simulink model "ModeAdjust"  (R2018b)
settings: Solver=FixedStepDiscrete  StartTime=0.0  StopTime=inf  FixedStep=0.01  RelTol=1e-3
undefined symbols (not defined in the file or in its folder): IfKeSMSbSeatMovBkRclnEnable_Val, IfKeSMSbSeatMovFrwdBkwdEnable_Val, IfKeSMSbSeatMovFtrstEnable_Val, IfKeSMSbSeatMovHdrstFrwdBkwdEnable_Val, IfKeSMSbSeatMovHdUpwdDnwdEnable_Val, IfKeSMSbSeatMovLgrstEnable_Val, IfKeSMSbSeatMovLtwdRtwdEnable_Val, IfVeSMSeStNumConfig, KeSMSbArmscreenMovEnable_Val, KeSMSbSeatMovLgrstExpdEnable_Val, KeSMSuFirstRwStBackPosDelta_Val, KeSMSuFirstRwStBackPosTolr_Val, KeSMSuFirstRwStCushFrntPosDelta_Val, KeSMSuFirstRwStCushFrntPosTolr_Val, KeSMSuFirstRwStCushRePosDelta_Val, KeSMSuFirstRwStCushRePosTolr_Val, KeSMSuFirstRwStFootrestPosDelta_Val, KeSMSuFirstRwStFootrestPosTolr_Val, KeSMSuFirstRwStFwdBkwdPosDelta_Val, KeSMSuFirstRwStFwdBkwdPosTolr_Val, KeSMSuMdMotFinshdTm_Val, KeSMSuMdRetryTm1_Val, KeSMSuModeReqDurgTm_Val, KeSMSuSecRwStArmTochPosDelta_Val, KeSMSuSecRwStArmTochPosTolr_Val, KeSMSuSecRwStBackPosDelta_Val, KeSMSuSecRwStBackPosTolr_Val, KeSMSuSecRwStFtrstUpwdDnwdPosDelta_Val, KeSMSuSecRwStFtrstUpwdDnwdPosTolr_Val, KeSMSuSecRwStFwdBkwdPosDelta_Val, KeSMSuSecRwStFwdBkwdPosTolr_Val, KeSMSuSecRwStHeadrestFwdBkwdPosDelta_Val, KeSMSuSecRwStHeadrestFwdBkwdPosTolr_Val, KeSMSuSecRwStHeadrestUpwdDwnwdPosDelta_Val, KeSMSuSecRwStHeadrestUpwdDwnwdPosTolr_Val, KeSMSuSecRwStLegrestInOutPosDelta_Val, KeSMSuSecRwStLegrestInOutPosTolr_Val, KeSMSuSecRwStLegrestUpwdDwnwdPosDelta_Val, KeSMSuSecRwStLegrestUpwdDwnwdPosTolr_Val, KeSMSuSecRwStLwdRwdPosDelta_Val, KeSMSuSecRwStLwdRwdPosTolr_Val, KeSMSuSecRwStVIPFtrstRefAngle_Val, KeSMSuThirdRwStFwdBkwdPosDelta_Val, KeSMSuThirdRwStFwdBkwdPosTolr_Val, KeSMSuThrdRwCushFoldPosDelta_Val, KeSMSuThrdRwCushFoldPosTolr_Val, KeSMSuThrdRwStBackPosDelta_Val, KeSMSuThrdRwStBackPosTolr_Val, KeSMSw4SLegrstCloseMdSecRwLtStFtrstUpwdDnwdPos_Val, KeSMSw4SLegrstCloseMdSecRwLtStFtrstUpwdDnwdPosMax_Val, KeSMSw4SLegrstCloseMdSecRwLtStFtrstUpwdDnwdPosMin_Val, KeSMSw4SLegrstCloseMdSecRwLtStLgrstOtwdInwdPos_Val, KeSMSw4SLegrstCloseMdSecRwLtStLgrstOtwdInwdPosMax_Val, KeSMSw4SLegrstCloseMdSecRwLtStLgrstOtwdInwdPosMin_Val, KeSMSw4SLegrstCloseMdSecRwLtStLgrstUpwdDnwdPos_Val, KeSMSw4SLegrstCloseMdSecRwLtStLgrstUpwdDnwdPosMax_Val, KeSMSw4SLegrstCloseMdSecRwLtStLgrstUpwdDnwdPosMin_Val, KeSMSw4SLegrstCloseMdSecRwRtStFtrstUpwdDnwdPos_Val, KeSMSw4SLegrstCloseMdSecRwRtStFtrstUpwdDnwdPosMax_Val, KeSMSw4SLegrstCloseMdSecRwRtStFtrstUpwdDnwdPosMin_Val ... (+1138)
libraries: Lib x401
(part 13 of 35)

== system ModeAdjust/ModeAdjustRunnable_sys/ModeAdjust/AcsMdExt/R2Lt ==
  note: %1锁，2未锁
  Mode_Trig : Inport
  Step1En : Inport  Port=2
  Step2En : Inport  Port=3
  SecRwLtStsPoss : Inport  Port=4
  SecRwLtStPossV : Inport  Port=5
  SecRwRtStChldLkRsp_L : Inport  Port=6
  ModeStCalib_2L : Inport  Port=7
  StConfig : Inport  Port=8
  isR2LtSeatOccupied : Inport  Port=9
  AND : Logic  AllPortsSameDT=off  OutDataTypeStr=boolean
  Bus Creator : BusCreator  Inputs=9  OutDataTypeStr=Bus: SecRwLfSeatPos
  Bus Selector : BusSelector  OutputSignals=IfVeSMSuSecRwLtStBkReclnUpwdDnwdPos_Val_read,IfVeSMSuSecRwLtStFrwdBkwdPos_Val_read,IfVeSMSuSecRwLtStHPassStUpwdDnwdPos_Val_read,IfVeSMSuSecRwLtStLgrstUpwdDnwdPos_Val_read,IfVeSMSuSecRwLtStLtwdRtwdPos_Val_read,IfVeSMSuSecRwLtStArmScrnPos_Val_read
  Bus Selector1 : BusSelector  OutputSignals=IfVeSMSuSecRwLtStBkReclnUpwdDnwdPosV_Val_read,IfVeSMSuSecRwLtStFrwdBkwdPosV_Val_read,IfVeSMSuSecRwLtStHPassStUpwdDnwdPosV_Val_read,IfVeSMSuSecRwLtStLgrstUpwdDnwdPosV_Val_read,IfVeSMSuSecRwLtStLtwdRtwdPosV_Val_read,IfVeSMSuSecRwLtStArmScrnPosV_Val_read
  Bus Selector2 : BusSelector  OutputSignals=ArmScrnPos,ArmScrnPosMax,ArmScrnPosMin,BkReclnUpwdDnwdPos,BkReclnUpwdDnwdPosMax,BkReclnUpwdDnwdPosMin,FrwdBkwdPos,FrwdBkwdPosMax,FrwdBkwdPosMin,HdrstUpwdPos,HdrstUpwdPosMax,HdrstUpwdPosMin,LgrstUpwdPos,LgrstUpwdPosMax,LgrstUpwdPosMin,LtwdRtwdPos,LtwdRtwdPosMax,LtwdRtwdPosMin
  Bus Selector3 : BusSelector  OutputSignals=AcsExtSecRwLtSt
  Bus Selector4 : BusSelector  OutputSignals=BkReclnUpwdDnwdMovConfig,ArmTouchMovConfig,FrwdBkwdMovConfig,LgrstUpwdMovConfig,LtwdRtwdMovConfig
  Logical Operator1 : Logic  Inputs=3  AllPortsSameDT=off  OutDataTypeStr=boolean
  Logical Operator2 : Logic  Inputs=3  AllPortsSameDT=off  OutDataTypeStr=boolean
  Logical Operator3 : Logic  AllPortsSameDT=off  OutDataTypeStr=boolean
  Logical Operator4 : Logic  AllPortsSameDT=off  OutDataTypeStr=boolean
  Logical Operator5 : Logic  Operator=OR  AllPortsSameDT=off  OutDataTypeStr=boolean
  Logical Operator6 : Logic  AllPortsSameDT=off  OutDataTypeStr=boolean
  NOT : Logic  Operator=NOT  AllPortsSameDT=off  OutDataTypeStr=boolean
  PA_KeSMSuMdMotFinshdTm_Val : Constant  Value=KeSMSuMdMotFinshdTm_Val
  PA_KeSMSuMdRetryTm1_Val : Constant  Value=KeSMSuMdRetryTm1_Val
  PA_KeSMSuModeReqDurgTm_Val : Constant  Value=KeSMSuModeReqDurgTm_Val
  PA_KeSMSuSecRwStArmTochPosDelta_Val : Constant  Value=KeSMSuSecRwStArmTochPosDelta_Val
  PA_KeSMSuSecRwStBackPosDelta_Val : Constant  Value=KeSMSuSecRwStBackPosDelta_Val
  PA_KeSMSuSecRwStFwdBkwdPosDelta_Val : Constant  Value=KeSMSuSecRwStFwdBkwdPosDelta_Val
  PA_KeSMSuSecRwStLegrestUpwdDwnwdPosDelta_Val : Constant  Value=KeSMSuSecRwStLegrestUpwdDwnwdPosDelta_Val
  PA_KeSMSuSecRwStLwdRwdPosDelta_Val : Constant  Value=KeSMSuSecRwStLwdRwdPosDelta_Val
  PA_KeSMSwDltTrgtPos_Val{1,4,7..11,16..17} (9 alike) : Constant  Value=0  OutDataTypeStr=boolean
  PA_KeSMSwDltTrgtPos_Val{3,6,12..15,18..21} (10 alike) : Constant  Value=KeSMSwPosInvalidVal_Val
  PA_KeSMSwDltTrgtPos_Val2 : Constant  Value=SeatChldLkSt.ChldLkSt_Unlock
  PA_KeSMSwDltTrgtPos_Val22 : Constant  Value=3  OutDataTypeStr=uint8
  PA_KeSMSwDltTrgtPos_Val23 : Constant  Value=2  OutDataTypeStr=uint8
  PA_KeSMSwDltTrgtPos_Val5 : Constant  OutDataTypeStr=boolean
  PA_KeSMSwSecRwLtStVIPCllsnPt_Val : Constant  Value=KeSMSwSecRwLtStVIPCllsnPt_Val
  R2LtStArmScrnPos_Step1 : Lib/CommonUsed  SystemSampleTime=-1
  R2LtSt_BkReclnUpwdDnwd_Step1 : Lib/CommonUsed  SystemSampleTime=-1
  R2LtSt_FrwdBkwd_Step2 : Lib/CommonUsed  SystemSampleTime=-1
  R2LtSt_LtwdRtwd_Step3 : Lib/CommonUsed  SystemSampleTime=-1
  Relational Operator : RelationalOperator  Operator=~=  OutDataTypeStr=boolean  RndMeth=Simplest
  Relational Operator1 : RelationalOperator  Operator=<=  OutDataTypeStr=boolean  RndMeth=Simplest
  Relational Operator2 : RelationalOperator  Operator=~=  OutDataTypeStr=boolean  RndMeth=Simplest
  SecRwLtStLgrstUpwd_Step1 : Lib/CommonUsed  SystemSampleTime=-1
  Switch : Switch  Criteria=u2 ~= 0
  R2Lt_Step1_Ini : Outport
  R2Lt_Step2_Ini : Outport  Port=2
  R2Lt_Step1_done : Outport  Port=3
  R2Lt_Step2_done : Outport  Port=4
  R2Lt_TrgtPoss : Outport  Port=5  VectorParamsAs1DForOutWhenUnconnected=on
  IfVeSMSuSecRwLtStRclCmdSrv_Val_writeRaw : Outport  Port=6
  R2Lt_SpdCtrl : Outport  Port=7
  wires:
  PA_KeSMSwDltTrgtPos_Val20/1 -> Bus Creator/4  "SecRwLtStCshnRrUpwdDnwdTrgtPos"
  [R2LtStFrwdBkwd_TarPos] -> Bus Creator/5  "SecRwLtStFrwdBkwdTrgtPos"
  [R2Lt_BkReclnUpwdDnwd_TarPos] -> Bus Creator/1  "SecRwLtStBkReclnUpwdDnwdTrgtPos"
  PA_KeSMSwDltTrgtPos_Val18/1 -> Bus Creator/2  "SecRwLtStBlstOtwdInwdTrgtPos"
  [R2LtSt_LtwdRtwd_TarPos] -> Bus Creator/8  "SecRwLtStLtwdRtwdTrgtPos"
  PA_KeSMSwDltTrgtPos_Val19/1 -> Bus Creator/3  "SecRwLtStCshnFrntUpwdDnwdTrgtPos"
  [R2Lt_LgrstUpwd_TarPos] -> Bus Creator/7  "SecRwLtStLgrstUpwdDnwdTrgtPos"
  Bus Creator/1 -> R2Lt_TrgtPoss/1
  PA_KeSMSwDltTrgtPos_Val21/1 -> Bus Creator/6  "SecRwLtStHdrstUpwdDnwdTrgtPos"
  R2LtSt_LtwdRtwd_Step3/2 -> [Step2_2_ArrivedTarPos]
  R2LtSt_FrwdBkwd_Step2/2 -> [Step2_1_ArrivedTarPos]
  Logical Operator4/1 -> R2Lt_Step2_done/1
  Logical Operator2/1 -> R2Lt_Step1_done/1
  Logical Operator6/1 -> R2Lt_Step2_Ini/1
  [LtwdRtwd_inidone_Step2] -> Logical Operator6/2
  [FrwdBkwd_inidone_Step2] -> Logical Operator6/1
  Logical Operator1/1 -> R2Lt_Step1_Ini/1
  [ArmScrn_Step1_ini] -> Logical Operator1/3
  [LgrstUpwd_Step1_ini] -> Logical Operator1/2
  [ReclnUpwdDnwd_Step1_ini] -> Logical Operator1/1
  PA_KeSMSwSecRwLtStVIPCllsnPt_Val/1 -> Relational Operator1/2
  Relational Operator1/1 -> Logical Operator5/2
  [SecRwLtStFrwdBkwdPos] -> Relational Operator1/1
  [Step2done_1] -> Logical Operator5/1
  Logical Operator5/1 -> Logical Operator3/1
  [Step2En] -> Logical Operator3/2
  Logical Operator3/1 -> R2LtSt_LtwdRtwd_Step3/2
  [Step2done_2] -> Logical Operator4/2
  [Step2done_1] -> Logical Operator4/1
  R2LtSt_LtwdRtwd_Step3/3 -> [R2LtSt_LtwdRtwd_TarPos]
  R2LtSt_LtwdRtwd_Step3/1 -> [LtwdRtwd_inidone_Step2]
  R2LtSt_LtwdRtwd_Step3/4 -> [Step2done_2]
  PA_KeSMSwDltTrgtPos_Val17/1 -> R2LtSt_LtwdRtwd_Step3/9
  [KeSMSuSecRwStLwdRwdPosDelta_Val] -> R2LtSt_LtwdRtwd_Step3/7
  [Tick] -> R2LtSt_LtwdRtwd_Step3/11
  PA_KeSMSwDltTrgtPos_Val14/1 -> R2LtSt_LtwdRtwd_Step3/10
  [Trig] -> R2LtSt_LtwdRtwd_Step3/1
  [SecRwLtStLtwdRtwdPosV] -> R2LtSt_LtwdRtwd_Step3/8
  [SecRwLtStLtwdRtwdPos] -> R2LtSt_LtwdRtwd_Step3/3
  [K_LtwdRtwdPosMin] -> R2LtSt_LtwdRtwd_Step3/4
  [K_LtwdRtwdPos] -> R2LtSt_LtwdRtwd_Step3/6
  [K_LtwdRtwdPosMax] -> R2LtSt_LtwdRtwd_Step3/5
  [Step1done_3] -> Logical Operator2/3
  [Step1done_2] -> Logical Operator2/2
  [Step1done_1] -> Logical Operator2/1
  PA_KeSMSwDltTrgtPos_Val10/1 -> R2LtStArmScrnPos_Step1/9
  [SecRwLtStArmScrnPosV] -> R2LtStArmScrnPos_Step1/8
  [KeSMSuSecRwStArmTochPosDelta_Val] -> R2LtStArmScrnPos_Step1/7
  [K_ArmScrnPos] -> R2LtStArmScrnPos_Step1/6
  [K_ArmScrnPosMin] -> R2LtStArmScrnPos_Step1/4
  [K_ArmScrnPosMax] -> R2LtStArmScrnPos_Step1/5
  [Tick] -> R2LtStArmScrnPos_Step1/11
  PA_KeSMSwDltTrgtPos_Val13/1 -> R2LtStArmScrnPos_Step1/10
  [SecRwLtStArmScrnPos] -> R2LtStArmScrnPos_Step1/3
  [Step1En] -> R2LtStArmScrnPos_Step1/2
  [Trig] -> R2LtStArmScrnPos_Step1/1
  SecRwLtStLgrstUpwd_Step1/4 -> [Step1done_2]
  SecRwLtStLgrstUpwd_Step1/3 -> [R2Lt_LgrstUpwd_TarPos]
  SecRwLtStLgrstUpwd_Step1/2 -> [Step1_2_ArrivedTarPos]
  SecRwLtStLgrstUpwd_Step1/1 -> [LgrstUpwd_Step1_ini]
  [Tick] -> SecRwLtStLgrstUpwd_Step1/11
  PA_KeSMSwDltTrgtPos_Val12/1 -> SecRwLtStLgrstUpwd_Step1/10
  PA_KeSMSwDltTrgtPos_Val11/1 -> SecRwLtStLgrstUpwd_Step1/9
  [SecRwLtStLgrstUpwdDnwdPosV] -> SecRwLtStLgrstUpwd_Step1/8
  [KeSMSuSecRwStLegrestUpwdDwnwdPosDelta_Val] -> SecRwLtStLgrstUpwd_Step1/7
  [SecRwLtStBkReclnUpwdDnwdPosV] -> R2LtSt_BkReclnUpwdDnwd_Step1/8
  [SecRwLtStLgrstUpwdDnwdPos] -> SecRwLtStLgrstUpwd_Step1/3
  [K_LgrstUpwdPos] -> SecRwLtStLgrstUpwd_Step1/6
  [K_LgrstUpwdPosMax] -> SecRwLtStLgrstUpwd_Step1/5
  [K_LgrstUpwdPosMin] -> SecRwLtStLgrstUpwd_Step1/4
  [Step1En] -> SecRwLtStLgrstUpwd_Step1/2
  [Trig] -> SecRwLtStLgrstUpwd_Step1/1
  Relational Operator/1 -> [ChildLocker]
  PA_KeSMSwDltTrgtPos_Val2/1 -> Relational Operator/2
  SecRwRtStChldLkRsp_L/1 -> Relational Operator/1
  Bus Selector/1 -> [SecRwLtStBkReclnUpwdDnwdPos]  "<IfVeSMSuSecRwLtStBkReclnUpwdDnwdPos_Val_read>"
  Bus Selector1/2 -> [SecRwLtStFrwdBkwdPosV]  "<IfVeSMSuSecRwLtStFrwdBkwdPosV_Val_read>"
  Bus Selector1/1 -> [SecRwLtStBkReclnUpwdDnwdPosV]  "<IfVeSMSuSecRwLtStBkReclnUpwdDnwdPosV_Val_read>"
  Bus Selector/2 -> [SecRwLtStFrwdBkwdPos]  "<IfVeSMSuSecRwLtStFrwdBkwdPos_Val_read>"
  Bus Selector/4 -> [SecRwLtStLgrstUpwdDnwdPos]  "<IfVeSMSuSecRwLtStLgrstUpwdDnwdPos_Val_read>"
  Bus Selector1/5 -> [SecRwLtStLtwdRtwdPosV]  "<IfVeSMSuSecRwLtStLtwdRtwdPosV_Val_read>"
  Bus Selector/3 -> [SecRwLtStHPassStUpwdDnwdPos]  "<IfVeSMSuSecRwLtStHPassStUpwdDnwdPos_Val_read>"
  SecRwLtStPossV/1 -> Bus Selector1/1
  Bus Selector1/4 -> [SecRwLtStLgrstUpwdDnwdPosV]  "<IfVeSMSuSecRwLtStLgrstUpwdDnwdPosV_Val_read>"
  SecRwLtStsPoss/1 -> Bus Selector/1
  Bus Selector/5 -> [SecRwLtStLtwdRtwdPos]  "<IfVeSMSuSecRwLtStLtwdRtwdPos_Val_read>"
  Bus Selector1/3 -> [SecRwLtStHPassStUpwdDnwdPosV]  "<IfVeSMSuSecRwLtStHPassStUpwdDnwdPosV_Val_read>"
  R2LtSt_FrwdBkwd_Step2/4 -> [Step2done_1]
  R2LtSt_FrwdBkwd_Step2/3 -> [R2LtStFrwdBkwd_TarPos]
  [Tick] -> R2LtSt_FrwdBkwd_Step2/11
  [Tick] -> R2LtSt_BkReclnUpwdDnwd_Step1/11
  PA_KeSMSwDltTrgtPos_Val6/1 -> R2LtSt_FrwdBkwd_Step2/10
  PA_KeSMSwDltTrgtPos_Val16/1 -> R2LtSt_FrwdBkwd_Step2/9
  [ChildLocker] -> R2LtSt_BkReclnUpwdDnwd_Step1/9
  [SecRwLtStFrwdBkwdPosV] -> R2LtSt_FrwdBkwd_Step2/8
  [K_FrwdBkwdPos] -> R2LtSt_FrwdBkwd_Step2/6
  [Step2En] -> R2LtSt_FrwdBkwd_Step2/2
  [Trig] -> R2LtSt_FrwdBkwd_Step2/1
  [Step1En] -> R2LtSt_BkReclnUpwdDnwd_Step1/2
  R2LtSt_BkReclnUpwdDnwd_Step1/4 -> [Step1done_1]
  R2LtSt_BkReclnUpwdDnwd_Step1/3 -> [R2Lt_BkReclnUpwdDnwd_TarPos]
  PA_KeSMSwDltTrgtPos_Val3/1 -> R2LtSt_BkReclnUpwdDnwd_Step1/10
  [K_BkReclnUpwdDnwdPos] -> R2LtSt_BkReclnUpwdDnwd_Step1/6
  [SecRwLtStBkReclnUpwdDnwdPos] -> R2LtSt_BkReclnUpwdDnwd_Step1/3
  R2LtSt_BkReclnUpwdDnwd_Step1/2 -> [Step1_1_ArrivedTarPos]
  [K_BkReclnUpwdDnwdPosMin] -> R2LtSt_BkReclnUpwdDnwd_Step1/4
  R2LtSt_FrwdBkwd_Step2/1 -> [FrwdBkwd_inidone_Step2]
  R2LtSt_BkReclnUpwdDnwd_Step1/1 -> [ReclnUpwdDnwd_Step1_ini]
  [K_FrwdBkwdPosMin] -> R2LtSt_FrwdBkwd_Step2/4
  [KeSMSuSecRwStFwdBkwdPosDelta_Val] -> R2LtSt_FrwdBkwd_Step2/7
  [K_FrwdBkwdPosMax] -> R2LtSt_FrwdBkwd_Step2/5
  [SecRwLtStFrwdBkwdPos] -> R2LtSt_FrwdBkwd_Step2/3
  [KeSMSuSecRwStBackPosDelta_Val] -> R2LtSt_BkReclnUpwdDnwd_Step1/7
  Mode_Trig/1 -> [Trig]
  [Trig] -> R2LtSt_BkReclnUpwdDnwd_Step1/1
  [K_BkReclnUpwdDnwdPosMax] -> R2LtSt_BkReclnUpwdDnwd_Step1/5
  Step1En/1 -> [Step1En]
  Step2En/1 -> [Step2En]
  PA_KeSMSwDltTrgtPos_Val5/1 -> IfVeSMSuSecRwLtStRclCmdSrv_Val_writeRaw/1
  PA_KeSMSuModeReqDurgTm_Val/1 -> [Tick]
  [SecRwLtStArmScrnTrgtPos] -> Bus Creator/9  "SecRwLtStArmScrnTrgtPos"
  R2LtStArmScrnPos_Step1/4 -> [Step1done_3]
  R2LtStArmScrnPos_Step1/3 -> [SecRwLtStArmScrnTrgtPos]
  R2LtStArmScrnPos_Step1/2 -> [Step1_3_ArrivedTarPos]
  R2LtStArmScrnPos_Step1/1 -> [ArmScrn_Step1_ini]
  PA_KeSMSuSecRwStBackPosDelta_Val/1 -> [KeSMSuSecRwStBackPosDelta_Val]
  PA_KeSMSuMdMotFinshdTm_Val/1 -> [KeSMSuMdMotFinshdTm_Val]
  PA_KeSMSuSecRwStFwdBkwdPosDelta_Val/1 -> [KeSMSuSecRwStFwdBkwdPosDelta_Val]
  PA_KeSMSuSecRwStLwdRwdPosDelta_Val/1 -> [KeSMSuSecRwStLwdRwdPosDelta_Val]
  PA_KeSMSuSecRwStArmTochPosDelta_Val/1 -> [KeSMSuSecRwStArmTochPosDelta_Val]
  PA_KeSMSuSecRwStLegrestUpwdDwnwdPosDelta_Val/1 -> [KeSMSuSecRwStLegrestUpwdDwnwdPosDelta_Val]
  [KeSMSuMdMotFinshdTm_Val] -> R2LtSt_BkReclnUpwdDnwd_Step1/12
  [KeSMSuMdMotFinshdTm_Val] -> SecRwLtStLgrstUpwd_Step1/12
  [KeSMSuMdMotFinshdTm_Val] -> R2LtStArmScrnPos_Step1/12
  [KeSMSuMdMotFinshdTm_Val] -> R2LtSt_FrwdBkwd_Step2/12
  [KeSMSuMdMotFinshdTm_Val] -> R2LtSt_LtwdRtwd_Step3/12
  Bus Selector/6 -> [SecRwLtStArmScrnPos]  "<IfVeSMSuSecRwLtStArmScrnPos_Val_read>"
  Bus Selector1/6 -> [SecRwLtStArmScrnPosV]  "<IfVeSMSuSecRwLtStArmScrnPosV_Val_read>"
  Bus Selector2/1 -> [K_ArmScrnPos]  "<ArmScrnPos>"
  Bus Selector2/18 -> [K_LtwdRtwdPosMin]  "<LtwdRtwdPosMin>"
  Bus Selector2/16 -> [K_LtwdRtwdPos]  "<LtwdRtwdPos>"
  Bus Selector2/15 -> [K_LgrstUpwdPosMin]  "<LgrstUpwdPosMin>"
  Bus Selector2/17 -> [K_LtwdRtwdPosMax]  "<LtwdRtwdPosMax>"
  Bus Selector2/12 -> [K_HdrstUpwdPosMin]  "<HdrstUpwdPosMin>"
  Bus Selector2/13 -> [K_LgrstUpwdPos]  "<LgrstUpwdPos>"
  Bus Selector2/11 -> [K_HdrstUpwdPosMax]  "<HdrstUpwdPosMax>"
  Bus Selector2/14 -> [K_LgrstUpwdPosMax]  "<LgrstUpwdPosMax>"
  Bus Selector2/10 -> [K_HdrstUpwdPos]  "<HdrstUpwdPos>"
  Bus Selector2/4 -> [K_BkReclnUpwdDnwdPos]  "<BkReclnUpwdDnwdPos>"
  Bus Selector2/9 -> [K_FrwdBkwdPosMin]  "<FrwdBkwdPosMin>"
  Bus Selector2/5 -> [K_BkReclnUpwdDnwdPosMax]  "<BkReclnUpwdDnwdPosMax>"
  Bus Selector2/8 -> [K_FrwdBkwdPosMax]  "<FrwdBkwdPosMax>"
  Bus Selector3/1 -> Bus Selector2/1  "<AcsExtSecRwLtSt>"
  Bus Selector2/7 -> [K_FrwdBkwdPos]  "<FrwdBkwdPos>"
  Bus Selector2/3 -> [K_ArmScrnPosMin]  "<ArmScrnPosMin>"
  Bus Selector2/2 -> [K_ArmScrnPosMax]  "<ArmScrnPosMax>"
  Bus Selector2/6 -> [K_BkReclnUpwdDnwdPosMin]  "<BkReclnUpwdDnwdPosMin>"
  ModeStCalib_2L/1 -> Bus Selector3/1
  PA_KeSMSwDltTrgtPos_Val1/1 -> R2LtSt_BkReclnUpwdDnwd_Step1/13
  PA_KeSMSwDltTrgtPos_Val4/1 -> SecRwLtStLgrstUpwd_Step1/13
  PA_KeSMSwDltTrgtPos_Val7/1 -> R2LtStArmScrnPos_Step1/13
  PA_KeSMSwDltTrgtPos_Val8/1 -> R2LtSt_FrwdBkwd_Step2/13
  PA_KeSMSwDltTrgtPos_Val9/1 -> R2LtSt_LtwdRtwd_Step3/13
  StConfig/1 -> Bus Selector4/1
  Bus Selector4/4 -> [LgrstUpwdMovConfig]  "<LgrstUpwdMovConfig>"
  Bus Selector4/3 -> [FrwdBkwdMovConfig]  "<FrwdBkwdMovConfig>"
  Bus Selector4/2 -> [ArmTouchMovConfig]  "<ArmTouchMovConfig>"
  Bus Selector4/1 -> [BkReclnUpwdDnwdMovConfig]  "<BkReclnUpwdDnwdMovConfig>"
  Bus Selector4/5 -> [LtwdRtwdMovConfig]  "<LtwdRtwdMovConfig>"
  [ArmTouchMovConfig] -> R2LtStArmScrnPos_Step1/14
  [LgrstUpwdMovConfig] -> SecRwLtStLgrstUpwd_Step1/14
  [LtwdRtwdMovConfig] -> R2LtSt_LtwdRtwd_Step3/14
  [FrwdBkwdMovConfig] -> R2LtSt_FrwdBkwd_Step2/14
  [BkReclnUpwdDnwdMovConfig] -> R2LtSt_BkReclnUpwdDnwd_Step1/14
  [CntLow] -> R2LtStArmScrnPos_Step1/15
  [CntLow] -> R2LtSt_BkReclnUpwdDnwd_Step1/15
  [CntLow] -> R2LtSt_FrwdBkwd_Step2/15
  [CntLow] -> R2LtSt_LtwdRtwd_Step3/15
  [CntLow] -> SecRwLtStLgrstUpwd_Step1/15
  PA_KeSMSuMdRetryTm1_Val/1 -> [CntLow]
  isR2LtSeatOccupied/1 -> NOT/1
  NOT/1 -> AND/1
  [R2LtStFrwdBkwd_TarPos] -> Relational Operator2/1  "SecRwLtStFrwdBkwdTrgtPos"
  PA_KeSMSwDltTrgtPos_Val15/1 -> Relational Operator2/2  "SecRwLtStHdrstUpwdDnwdTrgtPos"
  Relational Operator2/1 -> AND/2
  AND/1 -> Switch/2
  PA_KeSMSwDltTrgtPos_Val22/1 -> Switch/1
  PA_KeSMSwDltTrgtPos_Val23/1 -> Switch/3
  Switch/1 -> R2Lt_SpdCtrl/1

== system ModeAdjust/ModeAdjustRunnable_sys/ModeAdjust/AcsMdExt/R2Rt ==
  note: %1锁，2未锁
  Mode_Trig : Inport
  Step1En : Inport  Port=2
  Step2En : Inport  Port=3
  SecRwRtStPoss : Inport  Port=4
  SecRwRtStPossV : Inport  Port=5
  SecRwRtStChldLkRsp_L : Inport  Port=6
  ModeStCalib_2R : Inport  Port=7
  StConfig : Inport  Port=8
  isR2RtSeatOccupied : Inport  Port=9
  AND : Logic  AllPortsSameDT=off  OutDataTypeStr=boolean
  Bus Creator : BusCreator  Inputs=9  OutDataTypeStr=Bus: SecRwRtSeatPos
  Bus Selector : BusSelector  OutputSignals=IfVeSMSuSecRwRtStBkReclnUpwdDnwdPos_Val_read,IfVeSMSuSecRwRtStFrwdBkwdPos_Val_read,IfVeSMSuSecRwRtStHPassStUpwdDnwdPos_Val_read,IfVeSMSuSecRwRtStLgrstUpwdDnwdPos_Val_read,IfVeSMSuSecRwRtStLtwdRtwdPos_Val_read,SecRwRtStArmScrnPos_Val_read
  Bus Selector1 : BusSelector  OutputSignals=IfVeSMSuSecRwRtStBkReclnUpwdDnwdPosV_Val_read,IfVeSMSuSecRwRtStFrwdBkwdPosV_Val_read,IfVeSMSuSecRwRtStHPassStUpwdDnwdPosV_Val_read,IfVeSMSuSecRwRtStLgrstUpwdDnwdPosV_Val_read,IfVeSMSuSecRwRtStLtwdRtwdPosV_Val_read,SecRwRtStArmScrnPosV_Val_read
  Bus Selector2 : BusSelector  OutputSignals=ArmScrnPos,ArmScrnPosMax,ArmScrnPosMin,BkReclnUpwdDnwdPos,BkReclnUpwdDnwdPosMax,BkReclnUpwdDnwdPosMin,FrwdBkwdPos,FrwdBkwdPosMax,FrwdBkwdPosMin,HdrstUpwdPos,HdrstUpwdPosMax,HdrstUpwdPosMin,LgrstUpwdPos,LgrstUpwdPosMax,LgrstUpwdPosMin,LtwdRtwdPos,LtwdRtwdPosMax,LtwdRtwdPosMin
  Bus Selector3 : BusSelector  OutputSignals=AcsExtSecRwRSt
  Bus Selector4 : BusSelector  OutputSignals=BkReclnUpwdDnwdMovConfig,ArmTouchMovConfig,FrwdBkwdMovConfig,LgrstUpwdMovConfig,LtwdRtwdMovConfig
  Logical Operator1 : Logic  Inputs=3  AllPortsSameDT=off  OutDataTypeStr=boolean
  Logical Operator2 : Logic  Inputs=3  AllPortsSameDT=off  OutDataTypeStr=boolean
  Logical Operator3 : Logic  AllPortsSameDT=off  OutDataTypeStr=boolean
  Logical Operator4 : Logic  AllPortsSameDT=off  OutDataTypeStr=boolean
  Logical Operator5 : Logic  Operator=OR  AllPortsSameDT=off  OutDataTypeStr=boolean
  Logical Operator6 : Logic  AllPortsSameDT=off  OutDataTypeStr=boolean
  NOT : Logic  Operator=NOT  AllPortsSameDT=off  OutDataTypeStr=boolean
  PA_KeSMSuMdMotFinshdTm_Val : Constant  Value=KeSMSuMdMotFinshdTm_Val
  PA_KeSMSuMdRetryTm1_Val : Constant  Value=KeSMSuMdRetryTm1_Val
  PA_KeSMSuModeReqDurgTm_Val : Constant  Value=KeSMSuModeReqDurgTm_Val
  PA_KeSMSuSecRwStArmTochPosDelta_Val : Constant  Value=KeSMSuSecRwStArmTochPosDelta_Val
  PA_KeSMSuSecRwStBackPosDelta_Val : Constant  Value=KeSMSuSecRwStBackPosDelta_Val
  PA_KeSMSuSecRwStFwdBkwdPosDelta_Val : Constant  Value=KeSMSuSecRwStFwdBkwdPosDelta_Val
  PA_KeSMSuSecRwStLegrestUpwdDwnwdPosDelta_Val : Constant  Value=KeSMSuSecRwStLegrestUpwdDwnwdPosDelta_Val
  PA_KeSMSuSecRwStLwdRwdPosDelta_Val : Constant  Value=KeSMSuSecRwStLwdRwdPosDelta_Val
  PA_KeSMSwDltTrgtPos_Val{1,4..5,7..9,11,14,16} (9 alike) : Constant  Value=0  OutDataTypeStr=boolean
  PA_KeSMSwDltTrgtPos_Val{3,6,10,12,15,17,19..22} (10 alike) : Constant  Value=KeSMSwPosInvalidVal_Val
  PA_KeSMSwDltTrgtPos_Val18 : Constant  Value=3  OutDataTypeStr=uint8
  PA_KeSMSwDltTrgtPos_Val2 : Constant  Value=SeatChldLkSt.ChldLkSt_Unlock
  PA_KeSMSwDltTrgtPos_Val23 : Constant  OutDataTypeStr=boolean
  PA_KeSMSwDltTrgtPos_Val24 : Constant  Value=2  OutDataTypeStr=uint8
  PA_KeSMSwSecRwRtStVIPCllsnPt_Val : Constant  Value=KeSMSwSecRwRtStVIPCllsnPt_Val
  R2RtSt_ArmScrn_Step2 : Lib/CommonUsed  SystemSampleTime=-1
  R2RtSt_BkReclnUpwdDnwn_Step1 : Lib/CommonUsed  SystemSampleTime=-1
  R2RtSt_LgrstUpwd_Step1 : Lib/CommonUsed  SystemSampleTime=-1
  R2Rt_LtwdRtwd_Step2 : Lib/CommonUsed  SystemSampleTime=-1
  Relational Operator : RelationalOperator  Operator=~=  OutDataTypeStr=boolean  RndMeth=Simplest
  Relational Operator1 : RelationalOperator  Operator=<=  OutDataTypeStr=boolean  RndMeth=Simplest
  Relational Operator2 : RelationalOperator  Operator=~=  OutDataTypeStr=boolean  RndMeth=Simplest
  SecRwRtStFrwdBkwd_Step2 : Lib/CommonUsed  SystemSampleTime=-1
  Switch : Switch  Criteria=u2 ~= 0
  R2RtSt_Step1_ini : Outport
  R2RtSt_Step2_ini : Outport  Port=2
  R2Rt_Step1_done : Outport  Port=3
  R2Rt_Step2_done : Outport  Port=4
  R2Rt_TrgtPoss : Outport  Port=5  VectorParamsAs1DForOutWhenUnconnected=on
  IfVeSMSbSecRwRtStRclCmdSrv_Val_writeRaw : Outport  Port=6
  R2Rt_SpdCtrl : Outport  Port=7
  wires:
  PA_KeSMSwDltTrgtPos_Val21/1 -> Bus Creator/4  "SecRwRtStCshnRrUpwdDnwdTrgtPos"
  PA_KeSMSwDltTrgtPos_Val20/1 -> Bus Creator/3  "SecRwRtStCshnFrntUpwdDnwdTrgtPos"
  [R2RtSt_BkReclnUpwdDnwd_TarPos] -> Bus Creator/1  "SecRwRtStBkReclnUpwdDnwdTrgtPos"
  PA_KeSMSwDltTrgtPos_Val19/1 -> Bus Creator/2  "SecRwRtStBlstOtwdInwdTrgtPos"
  [R2RtSt_LgrstUpwd_TarPos] -> Bus Creator/7  "SecRwRtStLgrstUpwdDnwdTrgtPos"
  PA_KeSMSwDltTrgtPos_Val22/1 -> Bus Creator/6  "SecRwRtStHdrstUpwdDnwdTrgtPos"
  [R2Rt_LtwdRtwd_TarPos] -> Bus Creator/8  "SecRwRtStLtwdRtwdTrgtPos"
  [R2Rt_StFrwdBkwd_TarPos] -> Bus Creator/5  "SecRwRtStFrwdBkwdTrgtPos"
  Bus Creator/1 -> R2Rt_TrgtPoss/1
  Logical Operator3/1 -> R2Rt_Step2_done/1
  [Step2done_2] -> Logical Operator3/2
  [Step2done_1] -> Logical Operator3/1
  Logical Operator2/1 -> R2Rt_Step1_done/1
  Logical Operator6/1 -> R2RtSt_Step2_ini/1
  [LtwdRtwd_inidone_Step2] -> Logical Operator6/2
  [FrwdBkwd_inidone_Step2] -> Logical Operator6/1
  Logical Operator1/1 -> R2RtSt_Step1_ini/1
  [LtStArmScrn_Step1_ini] -> Logical Operator1/3
  [LgrstUpwd_Step1_ini] -> Logical Operator1/2
  [ReclnUpwdDnwd_Step1_ini] -> Logical Operator1/1
  R2RtSt_LgrstUpwd_Step1/1 -> [LgrstUpwd_Step1_ini]
  R2RtSt_BkReclnUpwdDnwn_Step1/1 -> [ReclnUpwdDnwd_Step1_ini]
  R2Rt_LtwdRtwd_Step2/4 -> [Step2done_2]
  R2Rt_LtwdRtwd_Step2/2 -> [Step2_2_ArrivedTarPos]
  R2Rt_LtwdRtwd_Step2/1 -> [LtwdRtwd_inidone_Step2]
  R2Rt_LtwdRtwd_Step2/3 -> [R2Rt_LtwdRtwd_TarPos]
  [Tick] -> R2Rt_LtwdRtwd_Step2/11
  PA_KeSMSwDltTrgtPos_Val17/1 -> R2Rt_LtwdRtwd_Step2/10
  PA_KeSMSwDltTrgtPos_Val16/1 -> R2Rt_LtwdRtwd_Step2/9
  [KeSMSuSecRwStLwdRwdPosDelta_Val] -> R2Rt_LtwdRtwd_Step2/7
  [K_LtwdRtwdPos] -> R2Rt_LtwdRtwd_Step2/6
  [K_LtwdRtwdPosMax] -> R2Rt_LtwdRtwd_Step2/5
  [K_LtwdRtwdPosMin] -> R2Rt_LtwdRtwd_Step2/4
  [SecRwRtStLtwdRtwdPosV] -> R2Rt_LtwdRtwd_Step2/8
  [SecRwRtStLtwdRtwdPos] -> R2Rt_LtwdRtwd_Step2/3
  [KeSMSuSecRwStArmTochPosDelta_Val] -> R2RtSt_ArmScrn_Step2/7
  [Step2En] -> Logical Operator4/2
  Relational Operator1/1 -> Logical Operator5/2
  Logical Operator4/1 -> R2Rt_LtwdRtwd_Step2/2
  Logical Operator5/1 -> Logical Operator4/1
  [Step2done_1] -> Logical Operator5/1
  [Trig] -> R2Rt_LtwdRtwd_Step2/1
  [SecRwRtStFrwdBkwdPos] -> Relational Operator1/1
  [Step1done_3] -> Logical Operator2/3
  [Step1done_2] -> Logical Operator2/2
  [Step1done_1] -> Logical Operator2/1
  SecRwRtStFrwdBkwd_Step2/3 -> [R2Rt_StFrwdBkwd_TarPos]
  [Tick] -> R2RtSt_ArmScrn_Step2/11
  PA_KeSMSwDltTrgtPos_Val10/1 -> R2RtSt_ArmScrn_Step2/10
  PA_KeSMSwDltTrgtPos_Val7/1 -> R2RtSt_ArmScrn_Step2/9
  [K_ArmScrnPos] -> R2RtSt_ArmScrn_Step2/6
  [K_ArmScrnPosMax] -> R2RtSt_ArmScrn_Step2/5
  [K_ArmScrnPosMin] -> R2RtSt_ArmScrn_Step2/4
  [Step1En] -> R2RtSt_ArmScrn_Step2/2
  [Trig] -> R2RtSt_ArmScrn_Step2/1
  [SecRwRtStArmScrnPosV] -> R2RtSt_ArmScrn_Step2/8
  [SecRwRtStArmScrnPos] -> R2RtSt_ArmScrn_Step2/3
  Bus Selector/2 -> [SecRwRtStFrwdBkwdPos]  "<IfVeSMSuSecRwRtStFrwdBkwdPos_Val_read>"
  Bus Selector/3 -> [SecRwRtStHPassStUpwdDnwdPos]  "<IfVeSMSuSecRwRtStHPassStUpwdDnwdPos_Val_read>"
  Bus Selector1/5 -> [SecRwRtStLtwdRtwdPosV]  "<IfVeSMSuSecRwRtStLtwdRtwdPosV_Val_read>"
  SecRwRtStPoss/1 -> Bus Selector/1
  Bus Selector/5 -> [SecRwRtStLtwdRtwdPos]  "<IfVeSMSuSecRwRtStLtwdRtwdPos_Val_read>"
  Bus Selector1/4 -> [SecRwRtStLgrstUpwdDnwdPosV]  "<IfVeSMSuSecRwRtStLgrstUpwdDnwdPosV_Val_read>"
  Bus Selector/1 -> [SecRwRtStBkReclnUpwdDnwdPos]  "<IfVeSMSuSecRwRtStBkReclnUpwdDnwdPos_Val_read>"
  Bus Selector1/1 -> [SecRwRtStBkReclnUpwdDnwdPosV]  "<IfVeSMSuSecRwRtStBkReclnUpwdDnwdPosV_Val_read>"
  Bus Selector/4 -> [SecRwRtStLgrstUpwdDnwdPos]  "<IfVeSMSuSecRwRtStLgrstUpwdDnwdPos_Val_read>"
  Bus Selector1/3 -> [SecRwRtStHPassStUpwdDnwdPosV]  "<IfVeSMSuSecRwRtStHPassStUpwdDnwdPosV_Val_read>"
  SecRwRtStPossV/1 -> Bus Selector1/1
  Bus Selector1/2 -> [SecRwRtStFrwdBkwdPosV]  "<IfVeSMSuSecRwRtStFrwdBkwdPosV_Val_read>"
  [K_BkReclnUpwdDnwdPosMax] -> R2RtSt_BkReclnUpwdDnwn_Step1/5
  [Trig] -> R2RtSt_BkReclnUpwdDnwn_Step1/1
  Mode_Trig/1 -> [Trig]
  [KeSMSuSecRwStBackPosDelta_Val] -> R2RtSt_BkReclnUpwdDnwn_Step1/7
  [SecRwRtStFrwdBkwdPos] -> SecRwRtStFrwdBkwd_Step2/3
  [K_FrwdBkwdPosMax] -> SecRwRtStFrwdBkwd_Step2/5
  [KeSMSuSecRwStFwdBkwdPosDelta_Val] -> SecRwRtStFrwdBkwd_Step2/7
  [K_FrwdBkwdPosMin] -> SecRwRtStFrwdBkwd_Step2/4
  SecRwRtStFrwdBkwd_Step2/1 -> [FrwdBkwd_inidone_Step2]
  SecRwRtStFrwdBkwd_Step2/2 -> [Step2_1_ArrivedTarPos]
  [K_BkReclnUpwdDnwdPosMin] -> R2RtSt_BkReclnUpwdDnwn_Step1/4
  R2RtSt_BkReclnUpwdDnwn_Step1/2 -> [Step1_1_ArrivedTarPos]
  [SecRwRtStBkReclnUpwdDnwdPos] -> R2RtSt_BkReclnUpwdDnwn_Step1/3
  [K_BkReclnUpwdDnwdPos] -> R2RtSt_BkReclnUpwdDnwn_Step1/6
  PA_KeSMSwDltTrgtPos_Val3/1 -> R2RtSt_BkReclnUpwdDnwn_Step1/10
  R2RtSt_BkReclnUpwdDnwn_Step1/3 -> [R2RtSt_BkReclnUpwdDnwd_TarPos]
  R2RtSt_BkReclnUpwdDnwn_Step1/4 -> [Step1done_1]
  [Step1En] -> R2RtSt_BkReclnUpwdDnwn_Step1/2
  [Trig] -> SecRwRtStFrwdBkwd_Step2/1
  [Step2En] -> SecRwRtStFrwdBkwd_Step2/2
  [K_FrwdBkwdPos] -> SecRwRtStFrwdBkwd_Step2/6
  [SecRwRtStFrwdBkwdPosV] -> SecRwRtStFrwdBkwd_Step2/8
  [ChildLocker] -> R2RtSt_BkReclnUpwdDnwn_Step1/9
  PA_KeSMSwDltTrgtPos_Val14/1 -> SecRwRtStFrwdBkwd_Step2/9
  PA_KeSMSwDltTrgtPos_Val6/1 -> SecRwRtStFrwdBkwd_Step2/10
  [Tick] -> R2RtSt_BkReclnUpwdDnwn_Step1/11
  [Tick] -> SecRwRtStFrwdBkwd_Step2/11
  SecRwRtStFrwdBkwd_Step2/4 -> [Step2done_1]
  SecRwRtStChldLkRsp_L/1 -> Relational Operator/1
  PA_KeSMSwDltTrgtPos_Val2/1 -> Relational Operator/2
  Relational Operator/1 -> [ChildLocker]
  [Trig] -> R2RtSt_LgrstUpwd_Step1/1
  [Step1En] -> R2RtSt_LgrstUpwd_Step1/2
  [K_LgrstUpwdPosMin] -> R2RtSt_LgrstUpwd_Step1/4
  [K_LgrstUpwdPosMax] -> R2RtSt_LgrstUpwd_Step1/5
  [K_LgrstUpwdPos] -> R2RtSt_LgrstUpwd_Step1/6
  [SecRwRtStLgrstUpwdDnwdPos] -> R2RtSt_LgrstUpwd_Step1/3
  [SecRwRtStBkReclnUpwdDnwdPosV] -> R2RtSt_BkReclnUpwdDnwn_Step1/8
  [KeSMSuSecRwStLegrestUpwdDwnwdPosDelta_Val] -> R2RtSt_LgrstUpwd_Step1/7
  [SecRwRtStLgrstUpwdDnwdPosV] -> R2RtSt_LgrstUpwd_Step1/8
  PA_KeSMSwDltTrgtPos_Val11/1 -> R2RtSt_LgrstUpwd_Step1/9
  PA_KeSMSwDltTrgtPos_Val12/1 -> R2RtSt_LgrstUpwd_Step1/10
  [Tick] -> R2RtSt_LgrstUpwd_Step1/11
  R2RtSt_LgrstUpwd_Step1/2 -> [Step1_2_ArrivedTarPos]
  R2RtSt_LgrstUpwd_Step1/3 -> [R2RtSt_LgrstUpwd_TarPos]
  R2RtSt_LgrstUpwd_Step1/4 -> [Step1done_2]
  PA_KeSMSwSecRwRtStVIPCllsnPt_Val/1 -> Relational Operator1/2
  Step1En/1 -> [Step1En]
  Step2En/1 -> [Step2En]
  PA_KeSMSwDltTrgtPos_Val23/1 -> IfVeSMSbSecRwRtStRclCmdSrv_Val_writeRaw/1
  PA_KeSMSuModeReqDurgTm_Val/1 -> [Tick]
  [SecRwRtStArmScrnTrgtPos] -> Bus Creator/9  "SecRwRtStArmScrnTrgtPos"
  R2RtSt_ArmScrn_Step2/1 -> [LtStArmScrn_Step1_ini]
  R2RtSt_ArmScrn_Step2/2 -> [Step1_3_ArrivedTarPos]
  R2RtSt_ArmScrn_Step2/3 -> [SecRwRtStArmScrnTrgtPos]
  R2RtSt_ArmScrn_Step2/4 -> [Step1done_3]
  PA_KeSMSuSecRwStBackPosDelta_Val/1 -> [KeSMSuSecRwStBackPosDelta_Val]
  PA_KeSMSuMdMotFinshdTm_Val/1 -> [KeSMSuMdMotFinshdTm_Val]
  PA_KeSMSuSecRwStFwdBkwdPosDelta_Val/1 -> [KeSMSuSecRwStFwdBkwdPosDelta_Val]
  PA_KeSMSuSecRwStLwdRwdPosDelta_Val/1 -> [KeSMSuSecRwStLwdRwdPosDelta_Val]
  PA_KeSMSuSecRwStArmTochPosDelta_Val/1 -> [KeSMSuSecRwStArmTochPosDelta_Val]
  PA_KeSMSuSecRwStLegrestUpwdDwnwdPosDelta_Val/1 -> [KeSMSuSecRwStLegrestUpwdDwnwdPosDelta_Val]
  [KeSMSuMdMotFinshdTm_Val] -> R2RtSt_BkReclnUpwdDnwn_Step1/12
  [KeSMSuMdMotFinshdTm_Val] -> R2RtSt_LgrstUpwd_Step1/12
  [KeSMSuMdMotFinshdTm_Val] -> R2RtSt_ArmScrn_Step2/12
  [KeSMSuMdMotFinshdTm_Val] -> SecRwRtStFrwdBkwd_Step2/12
  [KeSMSuMdMotFinshdTm_Val] -> R2Rt_LtwdRtwd_Step2/12
  Bus Selector/6 -> [SecRwRtStArmScrnPos]  "<SecRwRtStArmScrnPos_Val_read>"
  Bus Selector1/6 -> [SecRwRtStArmScrnPosV]  "<SecRwRtStArmScrnPosV_Val_read>"
  Bus Selector2/1 -> [K_ArmScrnPos]  "<ArmScrnPos>"
  Bus Selector2/18 -> [K_LtwdRtwdPosMin]  "<LtwdRtwdPosMin>"
  Bus Selector2/16 -> [K_LtwdRtwdPos]  "<LtwdRtwdPos>"
  Bus Selector2/15 -> [K_LgrstUpwdPosMin]  "<LgrstUpwdPosMin>"
  Bus Selector2/17 -> [K_LtwdRtwdPosMax]  "<LtwdRtwdPosMax>"
  Bus Selector2/12 -> [K_HdrstUpwdPosMin]  "<HdrstUpwdPosMin>"
  Bus Selector2/13 -> [K_LgrstUpwdPos]  "<LgrstUpwdPos>"
  Bus Selector2/11 -> [K_HdrstUpwdPosMax]  "<HdrstUpwdPosMax>"
  Bus Selector2/14 -> [K_LgrstUpwdPosMax]  "<LgrstUpwdPosMax>"
  Bus Selector2/10 -> [K_HdrstUpwdPos]  "<HdrstUpwdPos>"
  Bus Selector2/4 -> [K_BkReclnUpwdDnwdPos]  "<BkReclnUpwdDnwdPos>"
  Bus Selector2/9 -> [K_FrwdBkwdPosMin]  "<FrwdBkwdPosMin>"
  Bus Selector2/5 -> [K_BkReclnUpwdDnwdPosMax]  "<BkReclnUpwdDnwdPosMax>"
  Bus Selector2/8 -> [K_FrwdBkwdPosMax]  "<FrwdBkwdPosMax>"
  Bus Selector3/1 -> Bus Selector2/1  "<AcsExtSecRwRSt>"
  Bus Selector2/7 -> [K_FrwdBkwdPos]  "<FrwdBkwdPos>"
  Bus Selector2/3 -> [K_ArmScrnPosMin]  "<ArmScrnPosMin>"
  Bus Selector2/2 -> [K_ArmScrnPosMax]  "<ArmScrnPosMax>"
  Bus Selector2/6 -> [K_BkReclnUpwdDnwdPosMin]  "<BkReclnUpwdDnwdPosMin>"
  ModeStCalib_2R/1 -> Bus Selector3/1
  PA_KeSMSwDltTrgtPos_Val1/1 -> R2RtSt_BkReclnUpwdDnwn_Step1/13
  PA_KeSMSwDltTrgtPos_Val4/1 -> R2RtSt_LgrstUpwd_Step1/13
  PA_KeSMSwDltTrgtPos_Val5/1 -> R2RtSt_ArmScrn_Step2/13
  PA_KeSMSwDltTrgtPos_Val8/1 -> R2Rt_LtwdRtwd_Step2/13
  PA_KeSMSwDltTrgtPos_Val9/1 -> SecRwRtStFrwdBkwd_Step2/13
  StConfig/1 -> Bus Selector4/1
  Bus Selector4/4 -> [LgrstUpwdMovConfig]  "<LgrstUpwdMovConfig>"
  Bus Selector4/3 -> [FrwdBkwdMovConfig]  "<FrwdBkwdMovConfig>"
  Bus Selector4/2 -> [ArmTouchMovConfig]  "<ArmTouchMovConfig>"
  Bus Selector4/1 -> [BkReclnUpwdDnwdMovConfig]  "<BkReclnUpwdDnwdMovConfig>"
  Bus Selector4/5 -> [LtwdRtwdMovConfig]  "<LtwdRtwdMovConfig>"
  [BkReclnUpwdDnwdMovConfig] -> R2RtSt_BkReclnUpwdDnwn_Step1/14
  [LgrstUpwdMovConfig] -> R2RtSt_LgrstUpwd_Step1/14
  [FrwdBkwdMovConfig] -> SecRwRtStFrwdBkwd_Step2/14
  [LtwdRtwdMovConfig] -> R2Rt_LtwdRtwd_Step2/14
  [ArmTouchMovConfig] -> R2RtSt_ArmScrn_Step2/14
  [CntLow] -> R2RtSt_ArmScrn_Step2/15
  [CntLow] -> R2RtSt_BkReclnUpwdDnwn_Step1/15
  [CntLow] -> R2RtSt_LgrstUpwd_Step1/15
  [CntLow] -> R2Rt_LtwdRtwd_Step2/15
  [CntLow] -> SecRwRtStFrwdBkwd_Step2/15
  PA_KeSMSuMdRetryTm1_Val/1 -> [CntLow]
  [R2Rt_StFrwdBkwd_TarPos] -> Relational Operator2/1  "SecRwLtStFrwdBkwdTrgtPos"
  Switch/1 -> R2Rt_SpdCtrl/1
  PA_KeSMSwDltTrgtPos_Val18/1 -> Switch/1
  PA_KeSMSwDltTrgtPos_Val15/1 -> Relational Operator2/2  "SecRwLtStHdrstUpwdDnwdTrgtPos"
  AND/1 -> Switch/2
  isR2RtSeatOccupied/1 -> NOT/1
  NOT/1 -> AND/1
  Relational Operator2/1 -> AND/2
  PA_KeSMSwDltTrgtPos_Val24/1 -> Switch/3

== system ModeAdjust/ModeAdjustRunnable_sys/ModeAdjust/ArrivedAtTargetPosChk/AcsMdEntry ==
  DrvCurPos : Inport
  PassStPoss : Inport  Port=2
  SecRwLtStsPoss : Inport  Port=3
  SecRwRtStPoss : Inport  Port=4
  ThdRwLtStPoss : Inport  Port=5
  ThdRwRtStPoss : Inport  Port=6
  ModeStCalib : Inport  Port=7
  is6s : Inport  Port=8
  StConfig : Inport  Port=9
  DrvCurPosV : Inport  Port=10
  PassStPossV : Inport  Port=11
  SecRwLtStsPossV : Inport  Port=12
  SecRwRtStPossV : Inport  Port=13
  ThdRwLtStPossV : Inport  Port=14
  ThdRwRtStPossV : Inport  Port=15
  ChildLockerL : Inport  Port=16
  ChildLockerR : Inport  Port=17
  R3LOccupied : Inport  Port=18
  R3ROccupied : Inport  Port=19
  PosDeltaCalib : Inport  Port=20
  Bus Selector : BusSelector  OutputSignals=Calib_Drv,Calib_Pass,Calib_2L,Calib_2R,Calib_3L,Calib_3R
  Bus Selector1 : BusSelector  OutputSignals=DrvStConfig,PassStConfig,SecRwLtStConfig,SecRwRtStConfig,ThdRwLtStConfig,ThdRwRtStConfig
  Drv : Subsystem
  Logical Operator1 : Logic  Inputs=6  AllPortsSameDT=off  OutDataTypeStr=boolean
  Pass : Subsystem
  R2Lt : Subsystem
  R2Rt : Subsystem
  R3Lt : Subsystem
  R3Rt : Subsystem
  isAcsMdEntryArrivedAtTargetPos : Outport
  wires:
  [DrvST_ArrivedTarPos] -> Logical Operator1/1  "MdEntry_DrvST_ArrivedTarPos"
  Pass/1(Pass_ArrivedTarPos) -> [Pass_ArrivedTarPos]
  [Pass_ArrivedTarPos] -> Logical Operator1/2  "MdEntry_Pass_ArrivedTarPos"
  R2Lt/1(R2Lt_ArrivedTarPos) -> [R2LtST_ArrivedTarPos]
  [R2LtST_ArrivedTarPos] -> Logical Operator1/3  "MdEntry_R2LtST_ArrivedTarPos"
  R2Rt/1(R2Rt_ArrivedTarPos) -> [R2RtST_ArrivedTarPos]
  [R2RtST_ArrivedTarPos] -> Logical Operator1/4  "MdEntry_R2RtST_ArrivedTarPos"
  R3Lt/1(R3Lt_ArrivedTarPos) -> [R3LtST_ArrivedTarPos]
  [R3LtST_ArrivedTarPos] -> Logical Operator1/5  "MdEntry_R3LtST_ArrivedTarPos"
  R3Rt/1(R3Rt_ArrivedTarPos) -> [R3RtST_ArrivedTarPos]
  [R3RtST_ArrivedTarPos] -> Logical Operator1/6  "MdEntry_R3RtST_ArrivedTarPos"
  Logical Operator1/1 -> isAcsMdEntryArrivedAtTargetPos/1
  SecRwLtStsPoss/1 -> R2Lt/1(SecRwLtStsPoss)
  ThdRwLtStPoss/1 -> R3Lt/1(ThdRwLtStPoss)
  ThdRwRtStPoss/1 -> R3Rt/1(ThdRwRtStPoss)
  SecRwRtStPoss/1 -> R2Rt/1(SecRwRtStPoss)
  PassStPoss/1 -> Pass/1(PassStPoss)
  DrvCurPos/1 -> Drv/1(DrvCurPos)
  Drv/1(Drv_ArrivedTarPos) -> [DrvST_ArrivedTarPos]
  Bus Selector/6 -> [ModeStCalib_3R]  "<Calib_3R>"
  Bus Selector/4 -> [ModeStCalib_2R]  "<Calib_2R>"
  Bus Selector/1 -> [ModeStCalib_Drv]  "<Calib_Drv>"
  Bus Selector/3 -> [ModeStCalib_2L]  "<Calib_2L>"
  Bus Selector/5 -> [ModeStCalib_3L]  "<Calib_3L>"
  Bus Selector/2 -> [ModeStCalib_Pass]  "<Calib_Pass>"
  ModeStCalib/1 -> Bus Selector/1
  [ModeStCalib_Drv] -> Drv/2(ModeStCalib_Drv)
  [ModeStCalib_Pass] -> Pass/2(ModeStCalib_Pass)
  [ModeStCalib_2L] -> R2Lt/2(ModeStCalib_2L)
  [ModeStCalib_2R] -> R2Rt/2(ModeStCalib_2R)
  [ModeStCalib_3L] -> R3Lt/2(ModeStCalib_3L)
  [ModeStCalib_3R] -> R3Rt/2(ModeStCalib_3R)
  is6s/1 -> [is6s]
  [is6s] -> R3Lt/3(is6s)
  [is6s] -> R3Rt/3(is6s)
  Bus Selector1/6 -> [ThdRwRtStConfig]  "<ThdRwRtStConfig>"
  Bus Selector1/1 -> [DrvStConfig]  "<DrvStConfig>"
  Bus Selector1/3 -> [SecRwLtStConfig]  "<SecRwLtStConfig>"
  Bus Selector1/4 -> [SecRwRtStConfig]  "<SecRwRtStConfig>"
  StConfig/1 -> Bus Selector1/1
  Bus Selector1/2 -> [PassStConfig]  "<PassStConfig>"
  Bus Selector1/5 -> [ThdRwLtStConfig]  "<ThdRwLtStConfig>"
  [SecRwLtStConfig] -> R2Lt/3(StConfig)
  [DrvStConfig] -> Drv/3(StConfig)
  [PassStConfig] -> Pass/3(StConfig)
  [SecRwRtStConfig] -> R2Rt/3(StConfig)
  [ThdRwLtStConfig] -> R3Lt/4(StConfig)
  [ThdRwRtStConfig] -> R3Rt/4(StConfig)
  DrvCurPosV/1 -> Drv/4(DrvCurPosV)
  PassStPossV/1 -> Pass/4(PassStPossV)
  SecRwLtStsPossV/1 -> R2Lt/4(SecRwLtStPossV)
  ChildLockerL/1 -> R2Lt/5(ChildLockerL)
  SecRwRtStPossV/1 -> R2Rt/4(SecRwRtStPossV)
  ChildLockerR/1 -> R2Rt/5(ChildLockerR)
  ThdRwLtStPossV/1 -> R3Lt/5(ThdRwLtStPossV)
  R3LOccupied/1 -> R3Lt/6(R3LOccupied)
  ThdRwRtStPossV/1 -> R3Rt/5(ThdRwRtStPossV)
  R3ROccupied/1 -> R3Rt/6(R3ROccupied)
  PosDeltaCalib/1 -> [PosDeltaCalib]
  [PosDeltaCalib] -> Drv/5(PosDeltaCalib)
  [PosDeltaCalib] -> R2Lt/6(PosDeltaCalib)
  [PosDeltaCalib] -> R3Lt/7(PosDeltaCalib)
  [PosDeltaCalib] -> Pass/5(PosDeltaCalib)
  [PosDeltaCalib] -> R2Rt/6(PosDeltaCalib)
  [PosDeltaCalib] -> R3Rt/7(PosDeltaCalib)

== system ModeAdjust/ModeAdjustRunnable_sys/ModeAdjust/ArrivedAtTargetPosChk/AcsMdExt ==
  DrvCurPos : Inport
  PassStPoss : Inport  Port=2
  SecRwLtStsPoss : Inport  Port=3
  SecRwRtStPoss : Inport  Port=4
  ModeStCalib : Inport  Port=5
  StConfig : Inport  Port=6
  DrvCurPosV : Inport  Port=7
  PassStPossV : Inport  Port=8
  SecRwLtStsPossV : Inport  Port=9
  SecRwRtStPossV : Inport  Port=10
  ChildLockerL : Inport  Port=11
  ChildLockerR : Inport  Port=12
  PosDeltaCalib : Inport  Port=13
  Bus Selector : BusSelector  OutputSignals=Calib_Drv,Calib_Pass,Calib_2L,Calib_2R,Calib_3L,Calib_3R
  Bus Selector1 : BusSelector  OutputSignals=DrvStConfig,PassStConfig,SecRwLtStConfig,SecRwRtStConfig,ThdRwLtStConfig,ThdRwRtStConfig
  Drv : Subsystem
  Logical Operator1 : Logic  Inputs=4  AllPortsSameDT=off  OutDataTypeStr=boolean
  Pass : Subsystem
  R2Lt : Subsystem
  R2Rt : Subsystem
  isAcsMdExtArrivedAtTargetPos : Outport
  wires:
  SecRwRtStPoss/1 -> R2Rt/1(SecRwRtStPoss)
  SecRwLtStsPoss/1 -> R2Lt/1(SecRwLtStsPoss)
  PassStPoss/1 -> Pass/1(PassStPoss)
  DrvCurPos/1 -> Drv/1(DrvCurPos)
  Drv/1(Drv_ArrivedTarPos) -> [DrvST_ArrivedTarPos]
  Logical Operator1/1 -> isAcsMdExtArrivedAtTargetPos/1
  [R2RtST_ArrivedTarPos] -> Logical Operator1/4  "MdExt_R2RtST_ArrivedTarPos"
  R2Rt/1(R2Rt_ArrivedTarPos) -> [R2RtST_ArrivedTarPos]
  [R2LtST_ArrivedTarPos] -> Logical Operator1/3  "MdExt_R2LtST_ArrivedTarPos"
  [Pass_ArrivedTarPos] -> Logical Operator1/2  "MdExt_Pass_ArrivedTarPos"
  [DrvST_ArrivedTarPos] -> Logical Operator1/1  "MdExt_DrvST_ArrivedTarPos"
  Pass/1(Pass_ArrivedTarPos) -> [Pass_ArrivedTarPos]
  R2Lt/1(R2Lt_ArrivedTarPos) -> [R2LtST_ArrivedTarPos]
  Bus Selector/6 -> [ModeStCalib_3R]  "<Calib_3R>"
  Bus Selector/4 -> [ModeStCalib_2R]  "<Calib_2R>"
  Bus Selector/1 -> [ModeStCalib_Drv]  "<Calib_Drv>"
  Bus Selector/3 -> [ModeStCalib_2L]  "<Calib_2L>"
  Bus Selector/5 -> [ModeStCalib_3L]  "<Calib_3L>"
  Bus Selector/2 -> [ModeStCalib_Pass]  "<Calib_Pass>"
  ModeStCalib/1 -> Bus Selector/1
  [ModeStCalib_Drv] -> Drv/2(ModeStCalib_Drv)
  [ModeStCalib_Pass] -> Pass/2(ModeStCalib_Pass)
  [ModeStCalib_2L] -> R2Lt/2(ModeStCalib_2L)
  [ModeStCalib_2R] -> R2Rt/2(ModeStCalib_2R)
  Bus Selector1/6 -> [ThdRwRtStConfig]  "<ThdRwRtStConfig>"
  Bus Selector1/1 -> [DrvStConfig]  "<DrvStConfig>"
  Bus Selector1/3 -> [SecRwLtStConfig]  "<SecRwLtStConfig>"
  Bus Selector1/4 -> [SecRwRtStConfig]  "<SecRwRtStConfig>"
  StConfig/1 -> Bus Selector1/1
  Bus Selector1/2 -> [PassStConfig]  "<PassStConfig>"
  Bus Selector1/5 -> [ThdRwLtStConfig]  "<ThdRwLtStConfig>"
  [DrvStConfig] -> Drv/3(StConfig)
  [PassStConfig] -> Pass/3(StConfig)
  [SecRwLtStConfig] -> R2Lt/3(StConfig)
  [SecRwRtStConfig] -> R2Rt/3(StConfig)
  DrvCurPosV/1 -> Drv/4(DrvCurPosV)
  PassStPossV/1 -> Pass/4(PassStPossV)
  SecRwLtStsPossV/1 -> R2Lt/4(SecRwLtStPossV)
  ChildLockerL/1 -> R2Lt/5(ChildLockerL)
  SecRwRtStPossV/1 -> R2Rt/4(SecRwRtStPossV)
  ChildLockerR/1 -> R2Rt/5(ChildLockerR)
  PosDeltaCalib/1 -> [PosDeltaCalib]
  [PosDeltaCalib] -> Drv/5(PosDeltaCalib)
  [PosDeltaCalib] -> Pass/5(PosDeltaCalib)
  [PosDeltaCalib] -> R2Lt/6(PosDeltaCalib)
  [PosDeltaCalib] -> R2Rt/6(PosDeltaCalib)

== system ModeAdjust/ModeAdjustRunnable_sys/ModeAdjust/ArrivedAtTargetPosChk/Check4sHeight ==
  SecRwLtStsPoss : Inport
  Rev4sLEn : Inport  Port=2
  Ly4sLEn : Inport  Port=3
  VIP4sLEn : Inport  Port=4
  SecRwRtStPoss : Inport  Port=5
  Rev4sREn : Inport  Port=6
  Ly4sREn : Inport  Port=7
  VIP4sREn : Inport  Port=8
  4sLindex : Lib/Md4sHIghtindex  SystemSampleTime=-1
  4sRindex : Lib/Md4sHIghtindex  SystemSampleTime=-1
  Bus Selector : BusSelector  OutputSignals=IfVeSMSuSecRwLtStBkReclnUpwdDnwdPos_Val_read,IfVeSMSuSecRwLtStHPassStUpwdDnwdPos_Val_read
  Bus Selector1 : BusSelector  OutputSignals=IfVeSMSuSecRwRtStBkReclnUpwdDnwdPos_Val_read,IfVeSMSuSecRwRtStHPassStUpwdDnwdPos_Val_read
  Logical Operator : Logic  Operator=OR  Inputs=3  AllPortsSameDT=off  OutDataTypeStr=boolean
  Logical Operator1 : Logic  Operator=OR  Inputs=3  AllPortsSameDT=off  OutDataTypeStr=boolean
  Lt4sHightIndex : Outport
  Rt4sHightIndex : Outport  Port=2
  wires:
  4sLindex/1 -> Lt4sHightIndex/1
  SecRwRtStPoss/1 -> Bus Selector1/1
  Rev4sREn/1 -> Logical Operator/1
  Bus Selector/1 -> 4sLindex/1  "<IfVeSMSuSecRwLtStBkReclnUpwdDnwdPos_Val_read>"
  Logical Operator1/1 -> 4sLindex/3
  Logical Operator/1 -> 4sRindex/3
  Bus Selector/2 -> 4sLindex/2  "<IfVeSMSuSecRwLtStHPassStUpwdDnwdPos_Val_read>"
  Bus Selector1/1 -> 4sRindex/1  "<IfVeSMSuSecRwRtStBkReclnUpwdDnwdPos_Val_read>"
  Bus Selector1/2 -> 4sRindex/2  "<IfVeSMSuSecRwRtStHPassStUpwdDnwdPos_Val_read>"
  4sRindex/1 -> Rt4sHightIndex/1
  SecRwLtStsPoss/1 -> Bus Selector/1
  VIP4sREn/1 -> Logical Operator/3
  Rev4sLEn/1 -> Logical Operator1/1
  VIP4sLEn/1 -> Logical Operator1/3
  Ly4sREn/1 -> Logical Operator/2
  Ly4sLEn/1 -> Logical Operator1/2

== system ModeAdjust/ModeAdjustRunnable_sys/ModeAdjust/ArrivedAtTargetPosChk/FamlyL ==
  SecRwLtStsPoss : Inport
  SecRwRtStPoss : Inport  Port=2
  ThdRwRtStPoss : Inport  Port=3
  ModeStCalib : Inport  Port=4
  StConfig : Inport  Port=5
  SecRwLtStsPossV : Inport  Port=6
  SecRwRtStPossV : Inport  Port=7
  ThdRwRtStPossV : Inport  Port=8
  ThdRwLtStPoss : Inport  Port=9
  ThdRwLtStPossV : Inport  Port=10
  PosDeltaCalib : Inport  Port=11
  Bus Selector : BusSelector  OutputSignals=Calib_Drv,Calib_Pass,Calib_2L,Calib_2R,Calib_3L,Calib_3R
  Bus Selector1 : BusSelector  OutputSignals=DrvStConfig,PassStConfig,SecRwLtStConfig,SecRwRtStConfig,ThdRwLtStConfig,ThdRwRtStConfig
  Logical Operator1 : Logic  Inputs=4  AllPortsSameDT=off  OutDataTypeStr=boolean
  R2Lt : Subsystem
  R2Rt : Subsystem
  R3Lt : Subsystem
  R3Rt : Subsystem
  isLfFamlyArrivedAtTargetPos : Outport
  wires:
  [R3RtST_ArrivedTarPos] -> Logical Operator1/3
  [ThdRwRtStConfig] -> R3Rt/3(StConfig)
  [SecRwRtStConfig] -> R2Rt/3(StConfig)
  [SecRwLtStConfig] -> R2Lt/3(StConfig)
  Bus Selector1/5 -> [ThdRwLtStConfig]  "<ThdRwLtStConfig>"
  Bus Selector1/2 -> [PassStConfig]  "<PassStConfig>"
  StConfig/1 -> Bus Selector1/1
  Bus Selector1/4 -> [SecRwRtStConfig]  "<SecRwRtStConfig>"
  Bus Selector1/3 -> [SecRwLtStConfig]  "<SecRwLtStConfig>"
  Bus Selector1/1 -> [DrvStConfig]  "<DrvStConfig>"
  Bus Selector1/6 -> [ThdRwRtStConfig]  "<ThdRwRtStConfig>"
  [ModeStCalib_3R] -> R3Rt/2(ModeStCalib_3R)
  [ModeStCalib_2R] -> R2Rt/2(ModeStCalib_2R)
  [ModeStCalib_2L] -> R2Lt/2(ModeStCalib_2L)
  ModeStCalib/1 -> Bus Selector/1
  Bus Selector/2 -> [ModeStCalib_Pass]  "<Calib_Pass>"
  Bus Selector/5 -> [ModeStCalib_3L]  "<Calib_3L>"
  Bus Selector/3 -> [ModeStCalib_2L]  "<Calib_2L>"
  Bus Selector/1 -> [ModeStCalib_Drv]  "<Calib_Drv>"
  Bus Selector/4 -> [ModeStCalib_2R]  "<Calib_2R>"
  Bus Selector/6 -> [ModeStCalib_3R]  "<Calib_3R>"
  Logical Operator1/1 -> isLfFamlyArrivedAtTargetPos/1
  [R2RtST_ArrivedTarPos] -> Logical Operator1/2
  [R2LtST_ArrivedTarPos] -> Logical Operator1/1
  R2Lt/1(R2Lt_ArrivedTarPos) -> [R2LtST_ArrivedTarPos]
  R2Rt/1(R2Rt_ArrivedTarPos) -> [R2RtST_ArrivedTarPos]
  R3Rt/1(R3Rt_ArrivedTarPos) -> [R3RtST_ArrivedTarPos]
  SecRwLtStsPoss/1 -> R2Lt/1(SecRwLtStsPoss)
  ThdRwRtStPoss/1 -> R3Rt/1(ThdRwRtStPoss)
  SecRwRtStPoss/1 -> R2Rt/1(SecRwRtStPoss)
  SecRwLtStsPossV/1 -> R2Lt/4(SecRwLtStPossV)
  SecRwRtStPossV/1 -> R2Rt/4(SecRwRtStPossV)
  ThdRwRtStPossV/1 -> R3Rt/4(ThdRwRtStPossV)
  ThdRwLtStPossV/1 -> R3Lt/4(ThdRwLtStPossV)
  ThdRwLtStPoss/1 -> R3Lt/1(ThdRwLtStPoss)
  R3Lt/1(R3Lt_ArrivedTarPos) -> [R3LtST_ArrivedTarPos]
  [ModeStCalib_3L] -> R3Lt/2(ModeStCalib_3L)
  [ThdRwLtStConfig] -> R3Lt/3(StConfig)
  [R3LtST_ArrivedTarPos] -> Logical Operator1/4
  PosDeltaCalib/1 -> [PosDeltaCalib]
  [PosDeltaCalib] -> R2Lt/5(PosDeltaCalib)
  [PosDeltaCalib] -> R3Lt/5(PosDeltaCalib)
  [PosDeltaCalib] -> R2Rt/5(PosDeltaCalib)
  [PosDeltaCalib] -> R3Rt/5(PosDeltaCalib)

== system ModeAdjust/ModeAdjustRunnable_sys/ModeAdjust/ArrivedAtTargetPosChk/FamlyR ==
  SecRwLtStsPoss : Inport
  SecRwRtStPoss : Inport  Port=2
  ThdRwLtStPoss : Inport  Port=3
  ModeStCalib : Inport  Port=4
  StConfig : Inport  Port=5
  SecRwLtStsPossV : Inport  Port=6
  SecRwRtStPossV : Inport  Port=7
  ThdRwLtStPossV : Inport  Port=8
  ThdRwRtStPoss : Inport  Port=9
  ThdRwRtStPossV : Inport  Port=10
  PosDeltaCalib : Inport  Port=11
  Bus Selector : BusSelector  OutputSignals=Calib_Drv,Calib_Pass,Calib_2L,Calib_2R,Calib_3L,Calib_3R
  Bus Selector1 : BusSelector  OutputSignals=DrvStConfig,PassStConfig,SecRwLtStConfig,SecRwRtStConfig,ThdRwLtStConfig,ThdRwRtStConfig
  Logical Operator1 : Logic  Inputs=4  AllPortsSameDT=off  OutDataTypeStr=boolean
  R2Lt : Subsystem
  R2Rt : Subsystem
  R3Lt : Subsystem
  R3Rt : Subsystem
  isRtFamlyArrivedAtTargetPos : Outport
  wires:
  SecRwRtStPoss/1 -> R2Rt/1(SecRwRtStPoss)
  ThdRwLtStPoss/1 -> R3Lt/1(ThdRwLtStPoss)
  SecRwLtStsPoss/1 -> R2Lt/1(SecRwLtStsPoss)
  R3Lt/1(R3Lt_ArrivedTarPos) -> [R3LtST_ArrivedTarPos]
  R2Rt/1(R2Rt_ArrivedTarPos) -> [R2RtST_ArrivedTarPos]
  R2Lt/1(R2Lt_ArrivedTarPos) -> [R2LtST_ArrivedTarPos]
  [R2LtST_ArrivedTarPos] -> Logical Operator1/1
  Logical Operator1/1 -> isRtFamlyArrivedAtTargetPos/1
  Bus Selector/6 -> [ModeStCalib_3R]  "<Calib_3R>"
  Bus Selector/4 -> [ModeStCalib_2R]  "<Calib_2R>"
  Bus Selector/1 -> [ModeStCalib_Drv]  "<Calib_Drv>"
  Bus Selector/3 -> [ModeStCalib_2L]  "<Calib_2L>"
  Bus Selector/5 -> [ModeStCalib_3L]  "<Calib_3L>"
  Bus Selector/2 -> [ModeStCalib_Pass]  "<Calib_Pass>"
  ModeStCalib/1 -> Bus Selector/1
  [ModeStCalib_2L] -> R2Lt/2(ModeStCalib_2L)
  [ModeStCalib_2R] -> R2Rt/2(ModeStCalib_2R)
  [ModeStCalib_3L] -> R3Lt/2(ModeStCalib_3L)
  Bus Selector1/6 -> [ThdRwRtStConfig]  "<ThdRwRtStConfig>"
  Bus Selector1/1 -> [DrvStConfig]  "<DrvStConfig>"
  Bus Selector1/3 -> [SecRwLtStConfig]  "<SecRwLtStConfig>"
  Bus Selector1/4 -> [SecRwRtStConfig]  "<SecRwRtStConfig>"
  StConfig/1 -> Bus Selector1/1
  Bus Selector1/2 -> [PassStConfig]  "<PassStConfig>"
  Bus Selector1/5 -> [ThdRwLtStConfig]  "<ThdRwLtStConfig>"
  [SecRwLtStConfig] -> R2Lt/3(StConfig)
  [SecRwRtStConfig] -> R2Rt/3(StConfig)
  [ThdRwLtStConfig] -> R3Lt/3(StConfig)
  [R3LtST_ArrivedTarPos] -> Logical Operator1/3
  [R2RtST_ArrivedTarPos] -> Logical Operator1/2
  ThdRwLtStPossV/1 -> R3Lt/4(ThdRwLtStPossV)
  SecRwLtStsPossV/1 -> R2Lt/4(SecRwLtStPossV)
  SecRwRtStPossV/1 -> R2Rt/4(SecRwRtStPossV)
  ThdRwRtStPossV/1 -> R3Rt/4(ThdRwRtStPossV)
  ThdRwRtStPoss/1 -> R3Rt/1(ThdRwRtStPoss)
  R3Rt/1(R3Rt_ArrivedTarPos) -> [R3RtST_ArrivedTarPos]
  [ThdRwRtStConfig] -> R3Rt/3(StConfig)
  [ModeStCalib_3R] -> R3Rt/2(ModeStCalib_3R)
  [R3RtST_ArrivedTarPos] -> Logical Operator1/4
  PosDeltaCalib/1 -> [PosDeltaCalib]
  [PosDeltaCalib] -> R2Lt/5(PosDeltaCalib)
  [PosDeltaCalib] -> R2Rt/5(PosDeltaCalib)
  [PosDeltaCalib] -> R3Lt/5(PosDeltaCalib)
  [PosDeltaCalib] -> R3Rt/5(PosDeltaCalib)

== system ModeAdjust/ModeAdjustRunnable_sys/ModeAdjust/ArrivedAtTargetPosChk/INTML ==
  SecRwLtStsPoss : Inport
  SecRwRtStPoss : Inport  Port=2
  ModeStCalib : Inport  Port=3
  StConfig : Inport  Port=4
  SecRwLtStsPossV : Inport  Port=5
  SecRwRtStPossV : Inport  Port=6
  PosDeltaCalib : Inport  Port=7
  Bus Selector : BusSelector  OutputSignals=Calib_Drv,Calib_Pass,Calib_2L,Calib_2R,Calib_3L,Calib_3R
  Bus Selector1 : BusSelector  OutputSignals=DrvStConfig,PassStConfig,SecRwLtStConfig,SecRwRtStConfig,ThdRwLtStConfig,ThdRwRtStConfig
  Logical Operator : Logic  AllPortsSameDT=off  OutDataTypeStr=boolean
  R2Lt : Subsystem
  R2Rt : Subsystem
  isINTMArrivedAtTargetPos : Outport
  wires:
  [SecRwRtStConfig] -> R2Rt/3(StConfig)
  [SecRwLtStConfig] -> R2Lt/3(StConfig)
  Bus Selector1/5 -> [ThdRwLtStConfig]  "<ThdRwLtStConfig>"
  Bus Selector1/2 -> [PassStConfig]  "<PassStConfig>"
  StConfig/1 -> Bus Selector1/1
  Bus Selector1/4 -> [SecRwRtStConfig]  "<SecRwRtStConfig>"
  Bus Selector1/3 -> [SecRwLtStConfig]  "<SecRwLtStConfig>"
  Bus Selector1/1 -> [DrvStConfig]  "<DrvStConfig>"
  Bus Selector1/6 -> [ThdRwRtStConfig]  "<ThdRwRtStConfig>"
  [ModeStCalib_2L] -> R2Lt/2(ModeStCalib_2L)
  [ModeStCalib_2R] -> R2Rt/2(ModeStCalib_2R)
  ModeStCalib/1 -> Bus Selector/1
  Bus Selector/2 -> [ModeStCalib_Pass]  "<Calib_Pass>"
  Bus Selector/5 -> [ModeStCalib_3L]  "<Calib_3L>"
  Bus Selector/3 -> [ModeStCalib_2L]  "<Calib_2L>"
  Bus Selector/1 -> [ModeStCalib_Drv]  "<Calib_Drv>"
  Bus Selector/4 -> [ModeStCalib_2R]  "<Calib_2R>"
  Bus Selector/6 -> [ModeStCalib_3R]  "<Calib_3R>"
  SecRwRtStPoss/1 -> [SecRwRtStPoss], R2Rt/1(SecRwRtStPoss)
  SecRwLtStsPoss/1 -> R2Lt/1(SecRwLtStsPoss)
  R2Rt/1(R2Rt_ArrivedTarPos) -> [R2RtST_ArrivedTarPos]
  R2Lt/1(R2Lt_ArrivedTarPos) -> [R2LtST_ArrivedTarPos]
  Logical Operator/1 -> isINTMArrivedAtTargetPos/1
  [R2LtST_ArrivedTarPos] -> Logical Operator/1
  [R2RtST_ArrivedTarPos] -> Logical Operator/2
  SecRwLtStsPossV/1 -> R2Lt/4(SecRwLtStPossV)
  SecRwRtStPossV/1 -> R2Rt/4(SecRwRtStPossV)
  [SecRwRtStPoss] -> R2Lt/5(SecRwRtStPoss)
  PosDeltaCalib/1 -> [PosDeltaCalib]
  [PosDeltaCalib] -> R2Lt/6(PosDeltaCalib)
  [PosDeltaCalib] -> R2Rt/5(PosDeltaCalib)
